simulink library "KPIT_eBody_Lib_Lighting"  (R2022b)
settings: Solver=VariableStepAuto  StartTime=0.0  StopTime=10.0  RelTol=1e-3
undefined symbols (not defined in the file or in its folder): Float, Non, USAGEID_DEF, USAGEID_MIN
libraries: Alliance_Library x6
settings Model: Creator=smrithip1  LastModifiedBy=f064926

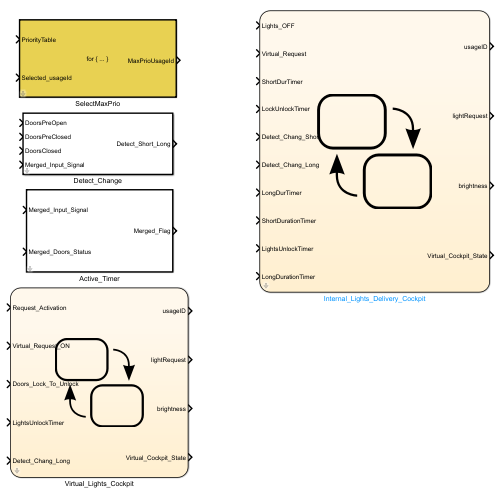
[thumbnail: Simulink's stored preview of the top-level diagram]
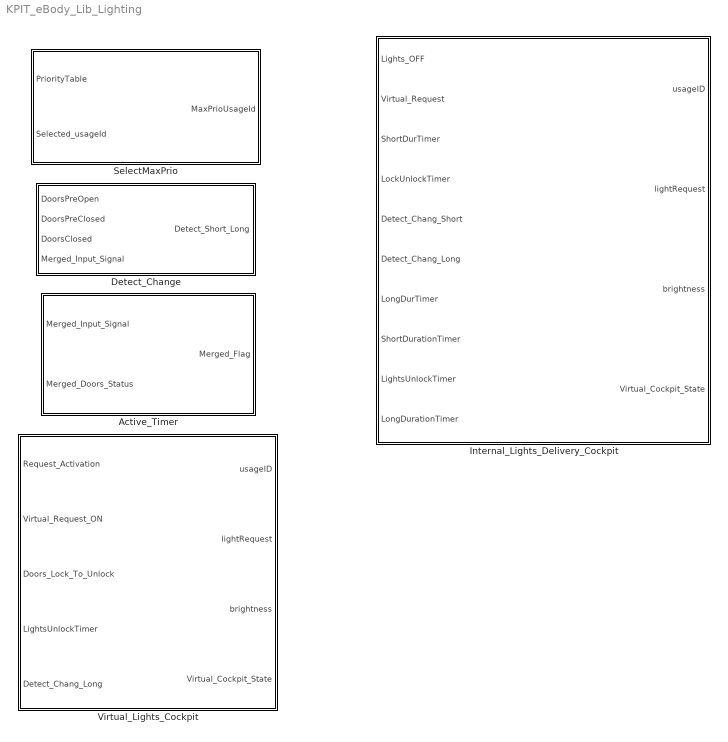
== system KPIT_eBody_Lib_Lighting ==
  Active_Timer : Subsystem  TreatAsAtomicUnit=on
      mask help: The subsystem Set the timer (Ramp Up and Ramp Down) as per the Vehicle power mode, Doors status and lock , unlock cabin doors
  Detect_Change : Subsystem  TreatAsAtomicUnit=on
      mask help:
      | Checking the  detect change of Light ON and Brightness
      | for reactive the subsystem
  Internal_Lights_Delivery_Cockpit : Stateflow chart  TreatAsAtomicUnit=on
      mask help:
      | Based on the VehiclePowerMode, doorStatus, Auto internal lights and Virtual internal lights inputs
      |  set the ouput for LightRequest and brightness
      settings: RTWSystemCode=Reusable function  PortSchema="{\"entries\":[{\"content\":{\"sides\":[{\"content\":{\"connectorIds\":[\"In3\",\"In6\",\"In7\",\"In8\",\"In4\",\"In5\",\"In2\",\"In9\",\"In10\",\"In1\"]},\"type\":\"ConnectorPlacement.EquallySpacedRectSide\",\"uuid\":\"fe5a48fb-f183-4d09-aaf2-298744077f7d\"},{\"content\":{\"connectorIds\":[\"Out3\",\"Out2\",\"Out1\",\"Out4\"],\"side\":\"RIGHT\"},\"type\":\"ConnectorPlacement.EquallySpacedRectSide\",\"uuid\":\"831a79d5-130d-4e2a-bce7-fe58e29d5782\"},{\"content\":{\"connectorIds\":[],\"side\":\"TOP\"},\"type\":\"ConnectorPlacement.EquallySpacedRectSide\",\"uuid\":\"a22c7bef-3a8a-471f-8360-1bf70d618e86\"},{\"content\":{\"connectorIds\":[],\"side\":\"BOTTOM\"},\"type\":\"ConnectorPlacement.EquallySpacedRectSide\",\"uuid\":\"0ad52087-765c-4138-b3c9-8ac1543edaf1\"}]},\"type\":\"ConnectorPlacement.EquallySpacedConnector\",\"uuid\":\"c594e464-93cd-4871-8c98-19cc5f98dd59\"}],\"packageUris\":[\"http://schema.mathworks.com/mf0/Connector/R2020b\"],\"version\":\"1.0\"}"
  SelectMaxPrio : Subsystem  Tag=[LIB]  mask(MaxPrioUsageId){}
      mask help:
      | Extracting the usage ID of the highest priority request
      |
      | Inputs:
      | 1. UsageID: Selected UsageID
      | 2. PriorityTable: Priority lookup table
      |
      | Outputs:
      | 1. MaxPrioUsageId: Usage ID of request with highest priority
      |
      | Constants:
      | PriorityTableLimit: Number of rows in the priority table (To be defined as a constant in the init.m file)
      | USAGEID_MIN: To be defined as 0 in init.m file
  Virtual_Lights_Cockpit : Stateflow chart  TreatAsAtomicUnit=on
      mask help: component will set Room Light Front and Rear and virtual cockpit state
      settings: RTWSystemCode=Reusable function  PortSchema="{\"entries\":[{\"content\":{\"sides\":[{\"content\":{\"connectorIds\":[\"In1\",\"In2\",\"In3\",\"In4\",\"In5\"]},\"type\":\"ConnectorPlacement.EquallySpacedRectSide\",\"uuid\":\"807e20c6-91e9-437a-a2ab-c0b73d38e528\"},{\"content\":{\"connectorIds\":[\"Out1\",\"Out3\",\"Out2\",\"Out4\"],\"side\":\"RIGHT\"},\"type\":\"ConnectorPlacement.EquallySpacedRectSide\",\"uuid\":\"dd64b57e-f041-47f7-9f0e-ae9d3ea9d5d0\"},{\"content\":{\"connectorIds\":[],\"side\":\"TOP\"},\"type\":\"ConnectorPlacement.EquallySpacedRectSide\",\"uuid\":\"cde97c66-9ec9-4740-b4d1-9b5a8ba137e8\"}]},\"type\":\"ConnectorPlacement.EquallySpacedConnector\",\"uuid\":\"2d72af5c-b9f1-4b2b-8de3-a9291656fcf5\"}],\"packageUris\":[\"http://schema.mathworks.com/mf0/Connector/R2020b\"],\"version\":\"1.0\"}"

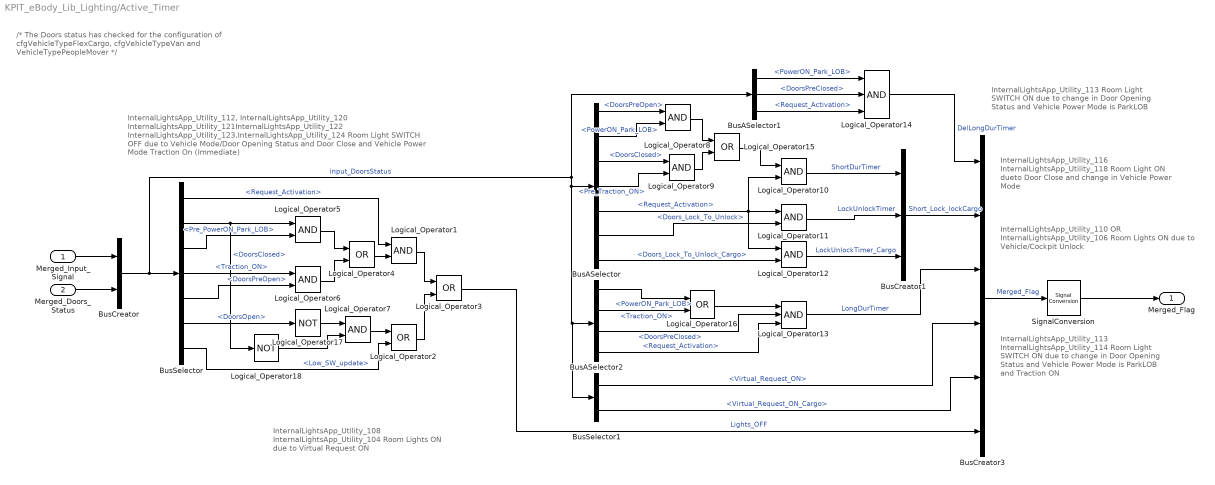
== system KPIT_eBody_Lib_Lighting/Active_Timer ==
  note: /* The Doors status has checked for the configuration of cfgVehicleTypeFlexCargo, cfgVehicleTypeVan and VehicleTypePeopleMover */
  note: InternalLightsApp_Utility_113
      | InternalLightsApp_Utility_114
      | Room Light SWITCH ON due
      | to change in Door Opening Status
      | and Vehicle Power Mode is ParkLOB
      | and Traction ON
  note: InternalLightsApp_Utility_116
      | InternalLightsApp_Utility_118
      | Room Light ON dueto Door Close
      | and change in Vehicle Power Mode
  note: InternalLightsApp_Utility_108
      | InternalLightsApp_Utility_104
      | Room Lights ON due to Virtual Request ON
  note: InternalLightsApp_Utility_110 OR
      | InternalLightsApp_Utility_106 Room
      | Lights ON due to Vehicle/Cockpit Unlock
  note: InternalLightsApp_Utility_112, InternalLightsApp_Utility_120
      | InternalLightsApp_Utility_121InternalLightsApp_Utility_122
      | InternalLightsApp_Utility_123,InternalLightsApp_Utility_124 Room Light SWITCH OFF due to Vehicle Mode/Door Opening Status and Door Close and Vehicle Power Mode Traction On (Immediate)
  note: InternalLightsApp_Utility_113
      | Room Light SWITCH ON due
      | to change in Door Opening Status
      | and Vehicle Power Mode is ParkLOB
  Merged_Input_Signal : Inport
  Merged_Doors_Status : Inport  Port=2
  BusASelector : BusSelector  OutputSignals=Merged_Doors_Status.DoorsPreOpen,Merged_Input_Signal.PowerON_Park_LOB,Merged_Doors_Status.DoorsClosed,Merged_Input_Signal.Pre_Traction_ON,Merged_Input_Signal.Request_Activation,Merged_Input_Signal.Doors_Lock_To_Unlock,Merged_Input_Signal.Doors_Lock_To_Unlock_Cargo
  BusASelector1 : BusSelector  OutputSignals=Merged_Input_Signal.PowerON_Park_LOB,Merged_Doors_Status.DoorsPreClosed,Merged_Input_Signal.Request_Activation
  BusASelector2 : BusSelector  OutputSignals=Merged_Input_Signal.PowerON_Park_LOB,Merged_Input_Signal.Traction_ON,Merged_Doors_Status.DoorsPreClosed,Merged_Input_Signal.Request_Activation
  BusCreator : BusCreator  Inputs=2
  BusCreator1 : BusCreator  Inputs=3
  BusCreator3 : BusCreator  Inputs=6
  BusSelector : BusSelector  OutputSignals=Merged_Input_Signal.Request_Activation,Merged_Doors_Status.DoorsClosed,Merged_Input_Signal.Pre_PowerON_Park_LOB,Merged_Input_Signal.Traction_ON,Merged_Doors_Status.DoorsPreOpen,Merged_Doors_Status.DoorsOpen,Merged_Input_Signal.Low_SW_update
  BusSelector1 : BusSelector  OutputSignals=Merged_Input_Signal.Virtual_Request_ON,Merged_Input_Signal.Virtual_Request_ON_Cargo
  Logical_Operator{1,5..12} (9 alike) : Logic  OutDataTypeStr=boolean
  Logical_Operator13 : Logic  Inputs=3  OutDataTypeStr=boolean
  Logical_Operator14 : Logic  Inputs=3  OutDataTypeStr=boolean
  Logical_Operator{2..4,15..16} (5 alike) : Logic  Operator=OR  OutDataTypeStr=boolean
  Logical_Operator17 : Logic  Operator=NOT  OutDataTypeStr=boolean
  Logical_Operator18 : Logic  Operator=NOT  OutDataTypeStr=boolean
  SignalConversion : SignalConversion  OverrideOpt=off
  Merged_Flag : Outport
  wires:
  Merged_Input_Signal/1 -> BusCreator/1
  Merged_Doors_Status/1 -> BusCreator/2
  BusCreator/1 -> BusSelector1/1, BusASelector2/1, BusASelector/1, BusASelector1/1, BusSelector/1  "input_DoorsStatus"
  BusSelector/1 -> Logical_Operator1/1  "<Request_Activation>"
  BusSelector/2 -> Logical_Operator18/1, Logical_Operator5/1  "<DoorsClosed>"
  BusSelector/3 -> Logical_Operator5/2  "<Pre_PowerON_Park_LOB>"
  BusSelector/4 -> Logical_Operator6/1  "<Traction_ON>"
  BusSelector/5 -> Logical_Operator6/2  "<DoorsPreOpen>"
  Logical_Operator5/1 -> Logical_Operator4/1
  Logical_Operator4/1 -> Logical_Operator1/2
  BusSelector/6 -> Logical_Operator17/1  "<DoorsOpen>"
  Logical_Operator18/1 -> Logical_Operator7/2
  BusSelector/7 -> Logical_Operator2/2  "<Low_SW_update>"
  Logical_Operator7/1 -> Logical_Operator2/1
  Logical_Operator1/1 -> Logical_Operator3/1
  Logical_Operator2/1 -> Logical_Operator3/2
  Logical_Operator3/1 -> BusCreator3/6  "Lights_OFF"
  BusASelector/1 -> Logical_Operator8/1  "<DoorsPreOpen>"
  BusASelector/2 -> Logical_Operator8/2  "<PowerON_Park_LOB>"
  BusASelector/3 -> Logical_Operator9/1  "<DoorsClosed>"
  BusASelector/4 -> Logical_Operator9/2  "<Pre_Traction_ON>"
  Logical_Operator8/1 -> Logical_Operator15/1
  Logical_Operator9/1 -> Logical_Operator15/2
  Logical_Operator15/1 -> Logical_Operator10/1
  BusASelector/5 -> Logical_Operator11/1, Logical_Operator10/2, Logical_Operator12/1  "<Request_Activation>"
  BusASelector2/1 -> Logical_Operator16/1  "<PowerON_Park_LOB>"
  BusASelector2/2 -> Logical_Operator16/2  "<Traction_ON>"
  Logical_Operator16/1 -> Logical_Operator13/1
  BusASelector2/3 -> Logical_Operator13/2  "<DoorsPreClosed>"
  BusASelector/6 -> Logical_Operator11/2  "<Doors_Lock_To_Unlock>"
  BusASelector2/4 -> Logical_Operator13/3  "<Request_Activation>"
  Logical_Operator10/1 -> BusCreator1/1  "ShortDurTimer"
  Logical_Operator11/1 -> BusCreator1/2  "LockUnlockTimer"
  Logical_Operator13/1 -> BusCreator3/3  "LongDurTimer"
  BusCreator1/1 -> BusCreator3/2  "Short_Lock_lockCargo"
  BusASelector/7 -> Logical_Operator12/2  "<Doors_Lock_To_Unlock_Cargo>"
  Logical_Operator12/1 -> BusCreator1/3  "LockUnlockTimer_Cargo"
  BusCreator3/1 -> SignalConversion/1  "Merged_Flag"
  BusASelector1/1 -> Logical_Operator14/1  "<PowerON_Park_LOB>"
  BusASelector1/2 -> Logical_Operator14/2  "<DoorsPreClosed>"
  BusASelector1/3 -> Logical_Operator14/3  "<Request_Activation>"
  Logical_Operator14/1 -> BusCreator3/1  "DelLongDurTimer"
  SignalConversion/1 -> Merged_Flag/1
  Logical_Operator17/1 -> Logical_Operator7/1
  Logical_Operator6/1 -> Logical_Operator4/2
  BusSelector1/1 -> BusCreator3/4  "<Virtual_Request_ON>"
  BusSelector1/2 -> BusCreator3/5  "<Virtual_Request_ON_Cargo>"

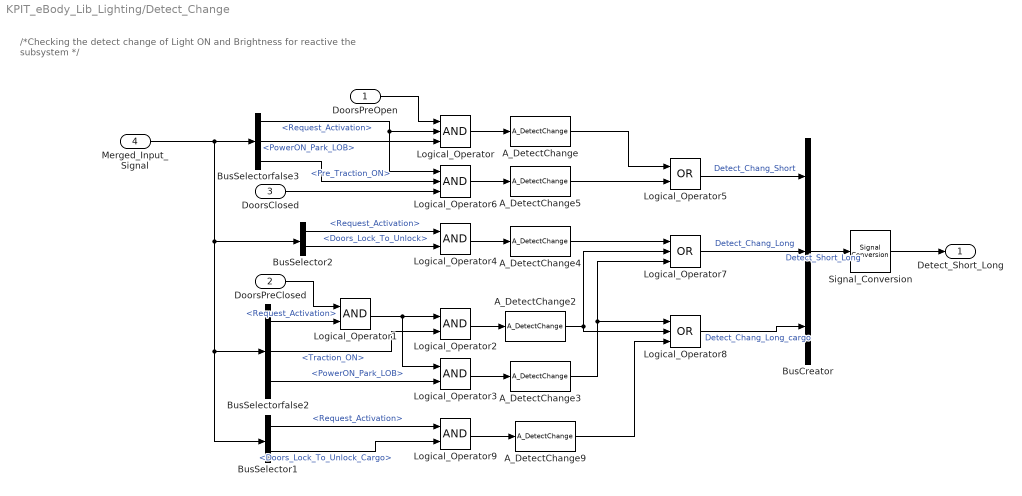
== system KPIT_eBody_Lib_Lighting/Detect_Change ==
  note: /*Checking the detect change of Light ON and Brightness
      | for reactive the subsystem */
  DoorsPreOpen : Inport
  DoorsPreClosed : Inport  Port=2
  DoorsClosed : Inport  Port=3
  Merged_Input_Signal : Inport  Port=4
  A_DetectChange{,2..5,9} (6 alike) : Alliance_Library/User_Defined_Libraries/Logic_and_Bit_Operations/A_DetectChange  Tag=[LIB]  LabelModeActiveChoice=NonFloat_CompInit  InputDataTyp=Non-Float  chkini=on  vinit=0  user_tol=eps
      settings: AttributesFormatString=|
      | %<MaskType>
      | DataType = %<InputDataTyp>
      | Comp with Init = %<chkini>
      | Initial Condition = %<vinit>
  BusCreator : BusCreator  Inputs=3
  BusSelector1 : BusSelector  OutputSignals=Request_Activation,Doors_Lock_To_Unlock_Cargo
  BusSelector2 : BusSelector  OutputSignals=Request_Activation,Doors_Lock_To_Unlock
  BusSelectorfalse2 : BusSelector  OutputSignals=Request_Activation,Traction_ON,PowerON_Park_LOB
  BusSelectorfalse3 : BusSelector  OutputSignals=Request_Activation,PowerON_Park_LOB,Pre_Traction_ON
  Logical_Operator : Logic  Inputs=3  OutDataTypeStr=boolean
  Logical_Operator{1..4,9} (5 alike) : Logic  OutDataTypeStr=boolean
  Logical_Operator5 : Logic  Operator=OR  OutDataTypeStr=boolean
  Logical_Operator6 : Logic  Inputs=3  OutDataTypeStr=boolean
  Logical_Operator7 : Logic  Operator=OR  Inputs=3  OutDataTypeStr=boolean
  Logical_Operator8 : Logic  Operator=OR  Inputs=3  OutDataTypeStr=boolean
  Signal_Conversion : SignalConversion  OverrideOpt=off
  Detect_Short_Long : Outport
  wires:
  DoorsPreOpen/1 -> Logical_Operator/1
  DoorsClosed/1 -> Logical_Operator6/3
  BusSelectorfalse3/1 -> Logical_Operator6/1, Logical_Operator/2  "<Request_Activation>"
  Logical_Operator/1 -> A_DetectChange/1
  BusSelectorfalse3/2 -> Logical_Operator/3  "<PowerON_Park_LOB>"
  Logical_Operator6/1 -> A_DetectChange5/1
  BusSelectorfalse3/3 -> Logical_Operator6/2  "<Pre_Traction_ON>"
  Logical_Operator5/1 -> BusCreator/1  "Detect_Chang_Short"
  A_DetectChange/1 -> Logical_Operator5/1
  A_DetectChange5/1 -> Logical_Operator5/2
  DoorsPreClosed/1 -> Logical_Operator1/1
  Logical_Operator1/1 -> Logical_Operator2/1, Logical_Operator3/1
  A_DetectChange3/1 -> Logical_Operator7/3, Logical_Operator8/1
  Logical_Operator3/1 -> A_DetectChange3/1
  Logical_Operator2/1 -> A_DetectChange2/1
  A_DetectChange2/1 -> Logical_Operator7/2, Logical_Operator8/2
  Logical_Operator4/1 -> A_DetectChange4/1
  BusSelectorfalse2/3 -> Logical_Operator3/2  "<PowerON_Park_LOB>"
  BusSelectorfalse2/2 -> Logical_Operator2/2  "<Traction_ON>"
  BusSelectorfalse2/1 -> Logical_Operator1/2  "<Request_Activation>"
  BusSelector2/1 -> Logical_Operator4/1  "<Request_Activation>"
  BusSelector2/2 -> Logical_Operator4/2  "<Doors_Lock_To_Unlock>"
  Logical_Operator7/1 -> BusCreator/2  "Detect_Chang_Long"
  BusCreator/1 -> Signal_Conversion/1  "Detect_Short_Long"
  A_DetectChange9/1 -> Logical_Operator8/3
  Logical_Operator9/1 -> A_DetectChange9/1
  Merged_Input_Signal/1 -> BusSelector1/1, BusSelectorfalse2/1, BusSelector2/1, BusSelectorfalse3/1
  BusSelector1/1 -> Logical_Operator9/1  "<Request_Activation>"
  BusSelector1/2 -> Logical_Operator9/2  "<Doors_Lock_To_Unlock_Cargo>"
  A_DetectChange4/1 -> Logical_Operator7/1
  Logical_Operator8/1 -> BusCreator/3  "Detect_Chang_Long_cargo"
  Signal_Conversion/1 -> Detect_Short_Long/1

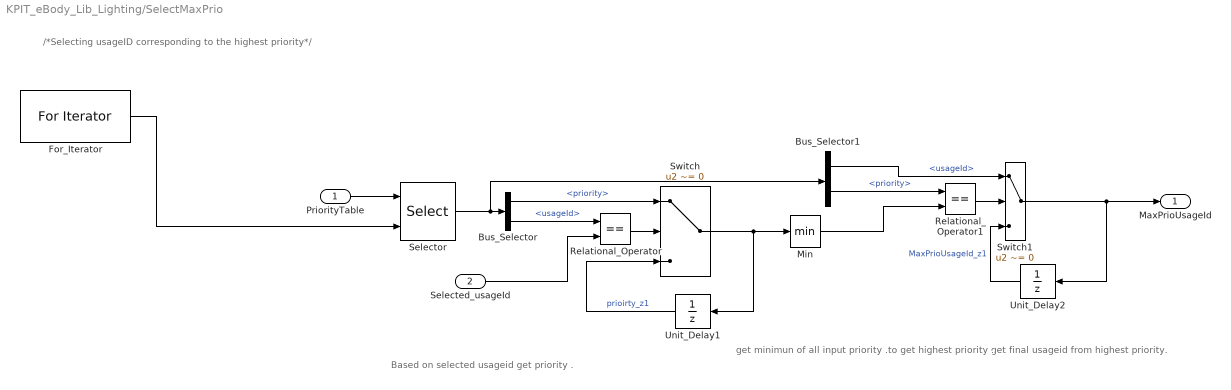
== system KPIT_eBody_Lib_Lighting/SelectMaxPrio ==
  note: /*Selecting usageID corresponding to the highest priority*/
  note: get final usageid from highest priority.
  note: get minimun of all input priority .to get highest priority .
  note: Based on selected usageid get priority .
  PriorityTable : Inport
  Selected_usageId : Inport  Port=2
  Bus_Selector : BusSelector  OutputSignals=priority,usageId
  Bus_Selector1 : BusSelector  OutputSignals=usageId,priority
  For_Iterator : ForIterator  ResetStates=reset  IterationLimit=PriorityTableLimit  IndexMode=Zero-based  IterationVariableDataType=uint8
      settings: AttributesFormatString=|
      | N = %<IterationLimit>
      | %<ResetStates>\n
  Min : MinMax  InputSameDT=on  RndMeth=Zero
  Relational_Operator : RelationalOperator  Operator===  OutDataTypeStr=boolean  RndMeth=Zero
  Relational_Operator1 : RelationalOperator  Operator===  OutDataTypeStr=boolean  RndMeth=Zero
  Selector : Selector  IndexMode=Zero-based  IndexOptions=Index vector (port)  Indices=[1 3]  OutputSizes=1
  Switch : Switch  Criteria=u2 ~= 0  RndMeth=Zero  SaturateOnIntegerOverflow=off
  Switch1 : Switch  Criteria=u2 ~= 0  RndMeth=Zero  SaturateOnIntegerOverflow=off
  Unit_Delay1 : UnitDelay  InitialCondition=USAGEID_DEF  SampleTime=-1  HasFrameUpgradeWarning=on
      settings: AttributesFormatString=Init = %<InitialCondition>
  Unit_Delay2 : UnitDelay  InitialCondition=USAGEID_MIN  SampleTime=-1  HasFrameUpgradeWarning=on
      settings: AttributesFormatString=Init = %<InitialCondition>
  MaxPrioUsageId : Outport
      settings: AttributesFormatString=Init = %<InitialOutput>\n
  wires:
  Relational_Operator1/1 -> Switch1/2
  Switch/1 -> Min/1, Unit_Delay1/1
  Relational_Operator/1 -> Switch/2
  Bus_Selector1/1 -> Switch1/1  "<usageId>"
  Min/1 -> Relational_Operator1/2
  Unit_Delay2/1 -> Switch1/3  "MaxPrioUsageId_z1"
  Selector/1 -> Bus_Selector1/1, Bus_Selector/1
  Bus_Selector1/2 -> Relational_Operator1/1  "<priority>"
  Bus_Selector/1 -> Switch/1  "<priority>"
  PriorityTable/1 -> Selector/1
  Unit_Delay1/1 -> Switch/3  "prioirty_z1"
  Selected_usageId/1 -> Relational_Operator/2
  Bus_Selector/2 -> Relational_Operator/1  "<usageId>"
  Switch1/1 -> Unit_Delay2/1, MaxPrioUsageId/1
  For_Iterator/1 -> Selector/2

== stateflow chart KPIT_eBody_Lib_Lighting/Internal_Lights_Delivery_Cockpit ==
  note: /*based on the VehiclePowerMode, doorOpeningStatus,
      | virtual cargo state , Auto internal lights inputs
      | set the ouput for LightRequest and brightness*/
  note: InternalLightsApp_Utility_110
      | InternalLightsApp_Utility_106
  note: InternalLightsApp_Utility_116
      | InternalLightsApp_Utility_118
  note: InternalLightsApp_Utility_113
      | InternalLightsApp_Utility_114
  note: InternalLightsApp_Utility_108
      | InternalLightsApp_Utility_104
  state DoNothing
    en:
    lightRequest = false;
    brightness= CONST_ZERO;
    Virtual_Cockpit_State =...
    INTERNALLIGHTSVIRTUALUSERSETTINGS_OFF
    usageID = CONST_ZERO;
  state Ramp_Up_Calculation
    en:
    Sample_Time = uint16(Ramp_Up_Time/TickTime);
    lightRequest = true;
    brightness = Min_Brightness;
    usageID = usageID_No;
    OFF_To_ON = false;
    Short_Du = false;
    Long_Du = false;
    state RampUp_LongDurationTimer
      en:
      LastValue = CONST_ZERO;
      countervalue = Min_Brightness;
      du:
      countervalue = countervalue+RamUp_CountTime;
      LastValue = countervalue;
      brightness = uint8(LastValue);
    state Ramp_UpTo_Ninety
      en:
      brightness = Full_Brightness;
      LastValue = Max_RampUp;
    (default) -> RampUp_LongDurationTimer
    RampUp_LongDurationTimer -> Ramp_UpTo_Ninety : [after((Sample_Time), tick)]
  note: InternalLightsApp_Utility_112, InternalLightsApp_Utility_120
      | InternalLightsApp_Utility_121InternalLightsApp_Utility_122
      | InternalLightsApp_Utility_123,InternalLightsApp_Utility_124
  state Ramp_Down_Calculation
    en:
    Virtual = false;
    Virtual_Cockpit_State = INTERNALLIGHTSVIRTUALUSERSETTINGS_OFF;
    Lock_Unlock = false;
    Short_T = false;
    state RampDown
      en:
      DownValue = LastValue;
      brightness = uint8(DownValue);
      du:
      DownValue = DownValue-RamDown_CountTime;
      brightness = uint8(DownValue);
    state RampDown_Upto_Zero
      en:
      lightRequest = false;
      brightness= CONST_ZERO;
      usageID = CONST_ZERO;
    (default) -> RampDown
    RampDown -> RampDown_Upto_Zero : [brightness <= Min_Brightness]
  note: InternalLightsApp_Utility_117InternalLightsApp_Utility_119
      | InternalLightsApp_Utility_109 Start the short Duration timer
  note: InternalLightsApp_Utility_115
      | Start the Long Duration timer start
  note: InternalLightsApp_Utility_111 Room
      | Light OFFdue to Door Open and Timer Expiry
  (default) -> (junction 239) : {lightRequest = false;
      | brightness = false;
      | usageID = CONST_ZERO;}
  (junction 239) -> DoNothing [order 4]
  (junction 363) -> (junction 235) [order 1] : [LongDurTimer]
  (junction 409) -> (junction 363) [order 2]
  (junction 239) -> (junction 409) [order 3]
  DoNothing -> (junction 239)
  (junction 239) -> Ramp_Up_Calculation [order 1] : [Virtual_Request]{Virtual = true;
      | Virtual_Cockpit_State =...
      |  INTERNALLIGHTSVIRTUALUSERSETTINGS_ON;}
  (junction 235) -> Ramp_Up_Calculation
  (junction 409) -> Ramp_Up_Calculation [order 1] : [ShortDurTimer]
      | {Short_T = true}
  (junction 239) -> (junction 276) [order 2]
  (junction 363) -> Ramp_Up_Calculation [order 2] : [LockUnlockTimer]
      | {Lock_Unlock = true;}
  (junction 435) -> Ramp_Up_Calculation : [LongDurTimer]
  (junction 432) -> (junction 435) [order 2]
  Ramp_Up_Calculation -> (junction 276) [order 2]
  (junction 276) -> Ramp_Down_Calculation : [Lights_OFF]...
      | {OFF_To_ON = true;}
  (junction 432) -> Ramp_Up_Calculation [order 1] : [LockUnlockTimer]
      | {Lock_Unlock = true;}
  (junction 366) -> (junction 432)
  Ramp_Up_Calculation -> (junction 281) [order 3]
  (junction 391) -> Ramp_Up_Calculation
  (junction 400) -> Ramp_Up_Calculation : [ShortDurTimer]
      | {Short_T = true}
  Ramp_Up_Calculation -> (junction 405) [order 1] : [(after((ShortDurationTimer/TickTime), tick) &&...
      | !Virtual_Request && Short_T) ||...
      | (!Virtual_Request && Virtual)]{Short_Du = true;}
  (junction 405) -> Ramp_Down_Calculation
  Ramp_Down_Calculation -> (junction 400) [order 3] : [OFF_To_ON || Long_Du || Detect_Chang_Short]
  Ramp_Down_Calculation -> (junction 391) [order 2] : [Virtual_Request]{Virtual_Cockpit_State = INTERNALLIGHTSVIRTUALUSERSETTINGS_ON}
  (junction 281) -> Ramp_Down_Calculation [order 1] : [(after(((LongDurationTimer)/TickTime), tick)...
      |  && !Virtual_Request)]{Long_Du = true;}
  (junction 281) -> (junction 322) [order 2]
  (junction 322) -> Ramp_Down_Calculation : [((after(((LightsUnlockTimer)/TickTime), tick)) &&...
      | Lock_Unlock && !Virtual_Request)]
      | {Long_Du = true;}
  Ramp_Down_Calculation -> (junction 366) [order 1] : [OFF_To_ON || Short_Du || Detect_Chang_Long]
  data: LongDurationTimer input uint16; LongDurTimer input; Lights_OFF input; brightness output Brightness =Brightnes; lightRequest output Enum: LightRequest =LightRequest.LIGHT_REQUEST_OFF; LastValue local single =Last_value; countervalue local single =CONST_zero; DownValue local single =CONST_zero; Sample_Time local uint16 =Sample_time; Full_Brightness constant uint8 =full_brightness; Max_RampUp constant uint8 =max_rampup; CONST_ZERO constant uint8 =CONST_zero; RamDown_CountTime constant single =RamDown_counttime; RamUp_CountTime constant single =RamUp_counttime; TickTime constant single =Tick_time; usageID output uint8 =ZERO; usageID_No constant uint8 =usageid_No; Ramp_Up_Time constant single =ram_up_time; Detect_Chang_Short input; Detect_Chang_Long input; Virtual local boolean =false; OFF_To_ON local boolean =false; Virtual_Cockpit_State output Enum: InternalLightsVirtualUserSettings =InternalLightsVirtualUserSettings.INTERNALLIGHTSVIRTUALUSERSETTINGS_OFF; Short_Du local boolean =false; Long_Du local boolean =false; Lock_Unlock local boolean =false; Short_T local boolean =false; Virtual_Request input; ShortDurTimer input; LockUnlockTimer input; ShortDurationTimer input uint8; LightsUnlockTimer input uint8; Min_Brightness constant uint8 =min_brightness

== stateflow chart KPIT_eBody_Lib_Lighting/Virtual_Lights_Cockpit ==
  note: /*Based on Auto internal lights App and Virtual light request input setting the out put of RoomLightFront and Virtual State*/
  note: /*Room Lights ON due to Vehicle/Cockpit Unlock InternalLightsApp_Utility_106
      | Unlock InternalLightsApp_Utility_110*/
  note: /*Room Lights ON due to Virtual Cockpit Request InternalLightsApp_Utility_104,InternalLightsApp_Utility_108*/
  state DoNothing
    //DoNothing
  state Ramp_Up_Calculation_ShortDuration
    en:
    Sample_Time = uint16(Ramp_Up_Time/TickTime);
    lightRequest = true;
    brightness = Min_Brightness;
    usageID = usageID_No;
    Virtual_Cockpit_State = INTERNALLIGHTSVIRTUALUSERSETTINGS_ON;
    state RampUp
      en:
      LastValue = CONST_ZERO;
      countervalue = Min_Brightness;
      du:
      countervalue = countervalue+RamUp_CountTime;
      LastValue = countervalue;
      brightness = uint8(LastValue);
    state RampUpTo_Ninety
      en:
      brightness = Full_Brightness;
      LastValue = Max_RampUp;
    (default) -> RampUp
    RampUp -> RampUpTo_Ninety : [after((Sample_Time), tick)]
  state Ramp_Up_Calculation
    en:
    Sample_Time = uint16(Ramp_Up_Time/TickTime);
    lightRequest = true;
    brightness = Min_Brightness;
    usageID = usageID_No;
    OFF_TO_NO = false;
    state RampUp_LongDuration
      en:
      LastValue = CONST_ZERO;
      countervalue = Min_Brightness;
      du:
      countervalue = countervalue+RamUp_CountTime;
      LastValue = countervalue;
      brightness = uint8(LastValue);
    state RampUp_Upto_Ninety
      en:
      brightness = Full_Brightness;
      LastValue = Max_RampUp;
    (default) -> RampUp_LongDuration
    RampUp_LongDuration -> RampUp_Upto_Ninety : [after((Sample_Time), tick)]
  note: /*Room Lights OFF due to Virtual Cockpit Request InternalLightsApp_Utility_105,InternalLightsApp_Utility_109*/
  note: /*Room Lights ON due to Vehicle/Cockpit Unlock InternalLightsApp_Utility_106*/
  note: Room Lights OFF due to Cockpit Unlock on Timer Expiry
      | InternalLightsApp_Utility_107
  state Ramp_Down_Calculation
    en:
    Virtual_Cockpit_State = INTERNALLIGHTSVIRTUALUSERSETTINGS_OFF;
    Lock_Unlock = false;
    state RampDown
      en:
      DownValue = LastValue;
      brightness = uint8(DownValue);
      du:
      DownValue = DownValue-RamDown_CountTime;
      brightness = uint8(DownValue);
    state RampDown_Upto_Zero
      en:
      lightRequest = false;
      brightness= CONST_ZERO;
      usageID = CONST_ZERO;
    (default) -> RampDown
    RampDown -> RampDown_Upto_Zero : [brightness <= Min_Brightness]
  (default) -> (junction 5) : {lightRequest = false;
      | brightness= CONST_ZERO;
      | usageID = CONST_ZERO;}
  (junction 5) -> (junction 41) [order 2] : [Request_Activation &&...
      |  Doors_Lock_To_Unlock ]
      | {Lock_Unlock = true}
  (junction 5) -> (junction 9) [order 1] : [Virtual_Request_ON]
  (junction 9) -> Ramp_Up_Calculation_ShortDuration
  (junction 5) -> DoNothing [order 4]
  DoNothing -> (junction 5)
  (junction 41) -> Ramp_Up_Calculation
  (junction 5) -> (junction 84) [order 3]
  Ramp_Up_Calculation_ShortDuration -> Ramp_Up_Calculation [order 2] : [Request_Activation &&...
      |  Doors_Lock_To_Unlock]
  Ramp_Up_Calculation -> (junction 84) [order 2]
  (junction 84) -> Ramp_Up_Calculation_ShortDuration [order 2] : [Virtual_Request_ON]
  (junction 84) -> Ramp_Down_Calculation [order 1] : [!Virtual_Request_ON &&...
      | !Lock_Unlock]
      | {OFF_TO_NO = true}
  Ramp_Down_Calculation -> Ramp_Up_Calculation_ShortDuration [order 1] : [Virtual_Request_ON]
  Ramp_Up_Calculation_ShortDuration -> Ramp_Down_Calculation [order 1] : [!Virtual_Request_ON]
  (junction 103) -> Ramp_Up_Calculation : [Request_Activation &&...
      |  Doors_Lock_To_Unlock &&...
      | (OFF_TO_NO || Detect_Chang_Long)]
      | {Lock_Unlock = true}
  Ramp_Up_Calculation -> (junction 105) [order 1] : [after((uint16(LightsUnlockTimer/TickTime)), tick)]
  (junction 105) -> Ramp_Down_Calculation
  Ramp_Down_Calculation -> (junction 103) [order 2]
  data: Request_Activation input; Virtual_Request_ON input boolean; Doors_Lock_To_Unlock input boolean; LightsUnlockTimer input uint8; usageID output uint8 =ZERO; TickTime constant single =Tick_time; RamDown_CountTime constant single =RamDown_counttime; RamUp_CountTime constant single =RamUp_counttime; CONST_ZERO constant uint8 =ZERO; Min_Brightness constant uint8 =min_brightness; Full_Brightness constant uint8 =full_brightness; Sample_Time local single =CONST_zero; Max_RampUp constant uint8 =max_rampup; DownValue local single =CONST_zero; countervalue local single =CONST_zero; LastValue local single =CONST_zero; brightness output uint8 =Brightnes; lightRequest output Enum: LightRequest =LightRequest.LIGHT_REQUEST_OFF; Virtual_Cockpit_State output Enum: InternalLightsVirtualUserSettings =InternalLightsVirtualUserSettings.INTERNALLIGHTSVIRTUALUSERSETTINGS_OFF; usageID_No constant uint8 =usageid_No; Detect_Chang_Long input; OFF_TO_NO local boolean =CONST_zero; Lock_Unlock local boolean =CONST_zero; Ramp_Up_Time constant single =ram_up_time
